simulink model "HW3_prob3"  (Simulink 7.8)
settings: Solver=ode45  StartTime=0.0  StopTime=1  MaxStep=.0005  RelTol=1e-3
values from neighbouring files (symbols this model uses):
  c = 1000    [Schur_HW1.m]    (also in Schur_HW10.m = [.05 .2  .5  1  5 20 50]; Schur_HW11.m = [.1 1 10 100 1000 10000]; Schur_HW3.m = 4000; Schur_HW4.m = zeta*2*sqrt(m*k1))
  k = 5000    [Schur_HW1.m]    (also in Schur_HW10.m = 25; Schur_HW11.m = wn.^2*m; Schur_HW12.m = 20000; Schur_HW2.m = 30000)
  Kp = -4.5*10^6    (= -4500000)    [Schur_HW3.m]    (also in week3_transfer_function.m)
  Kv = 0    [Schur_HW3.m]
  m = 10    [Schur_HW1.m]    (also in Schur_HW10.m = 1; Schur_HW11.m = 5; Schur_HW12.m = 100; Schur_HW2.m = 100)
  T = (M/(17/16*m*l^2))*(s^2/(s^2+w^2))*(1/(s^2+250*s+5000))    [Schur_HW1.m]    (also in Schur_HW3.m = [.01 .1 1 10 100]; Schur_HW6.m = 10)
settings Model: Creator=rschur  LastModifiedBy=Randy Schur
settings DataIOCC: SignalLoggingSaveFormat=Dataset
settings OptimizationCC: ExpressionDepthLimit=128
settings DebuggingCC: UnderspecifiedInitializationDetection=Simplified  MergeDetectMultiDrivingBlocksExec=error  StateNameClashWarn=none
settings CodeAppCC: CustomSymbolStrType=$N$R$M_T
settings GRTTargetCC: TargetFunctionLibrary=NOT IN USE  CombineOutputUpdateFcns=on  CPPClassGenCompliant=on

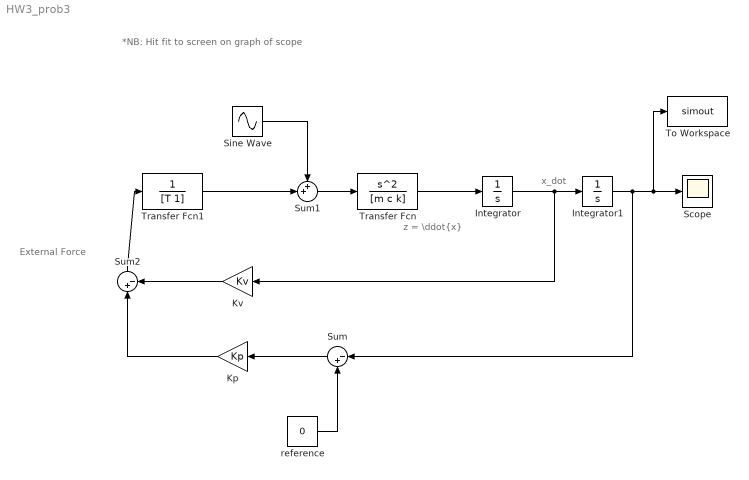
== system HW3_prob3 ==
  note: *NB: Hit fit to screen on graph of scope
  note: External Force
  note: x_dot
  note: z = \ddot{x}
  Integrator : Integrator
  Integrator1 : Integrator
  Kp : Gain  Gain=Kp
  Kv : Gain  Gain=Kv
  Scope : Scope
      settings: DataFormat=Array
  Sine Wave : Sin  Amplitude=100  Frequency=30*2*pi  SampleTime=0
  Sum : Sum  Inputs=|-+
  Sum1 : Sum  Inputs=++|
  Sum2 : Sum  Inputs=|+-
  To Workspace : ToWorkspace  VariableName=simout  SampleTime=-1  SaveFormat=Structure With Time
  Transfer Fcn : TransferFcn  Numerator=[1 0 0]  Denominator=[m c k]
  Transfer Fcn1 : TransferFcn  Denominator=[T 1]
  reference : Constant  Value=0
  wires:
  Transfer Fcn/1 -> Integrator/1
  Integrator/1 -> Kv/1, Integrator1/1
  reference/1 -> Sum/2
  Sum/1 -> Kp/1
  Sine Wave/1 -> Sum1/1
  Kv/1 -> Sum2/2
  Kp/1 -> Sum2/1
  Integrator1/1 -> To Workspace/1, Scope/1, Sum/1
  Sum2/1 -> Transfer Fcn1/1
  Transfer Fcn1/1 -> Sum1/2
  Sum1/1 -> Transfer Fcn/1
